simulink model "Cascata_piu_anelli"  (R2023b)
settings: Solver=VariableStepAuto  StartTime=0.0  StopTime=4  RelTol=1e-3
values from neighbouring files (symbols this model uses):
  den = [1 437.9395]    [controllore_piu_anelli.m]
  den_ext = [1 0]    [controllore_piu_anelli.m]
  Gdclose = Gdclose{1}    [controllore_piu_anelli.m]
  Gden = Gden{1}    [controllore_piu_anelli.m]
  Gnclose = Gnclose{1}    [controllore_piu_anelli.m]
  Gnum = Gnum{1}    [controllore_piu_anelli.m]
  num = [916.9165 8.0682e+04]    [controllore_piu_anelli.m]
  num_ext = [0.0081249 23.37*0.0081249]    [controllore_piu_anelli.m]
  ueq = 15/Rtot    [controllore_piu_anelli.m]
  x1_eq = 0.0044    [Controllo_un_anello_v2.m]    (also in Controllore_testato.m)
undefined symbols (not defined in the file or in its folder): ki, kp, Lc, Rtot
libraries: slpidlib x3
settings Model: Creator=lollo  LastModifiedBy=lollo

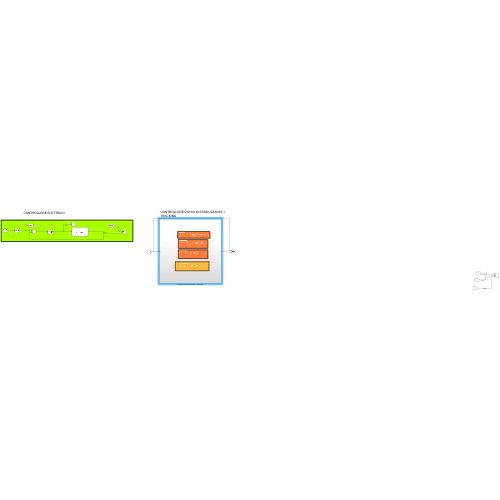
[thumbnail: Simulink's stored preview of the top-level diagram]
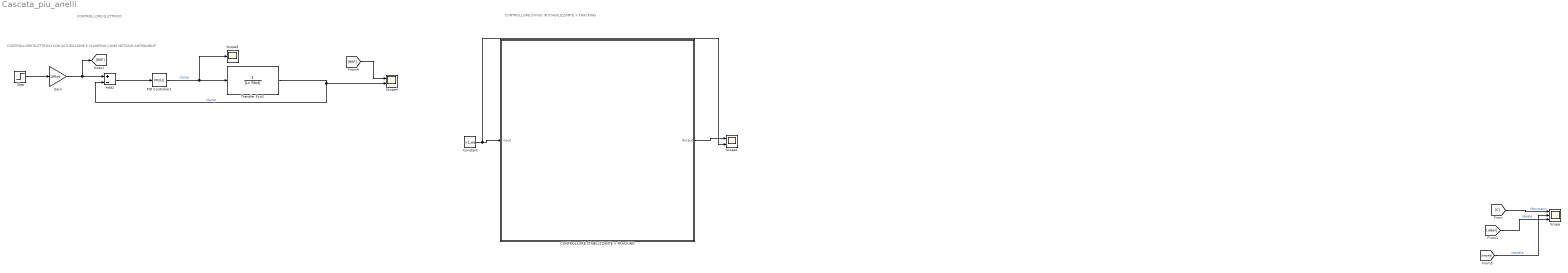
== system Cascata_piu_anelli ==
  note: CONTROLLORE ELETTRICO
  note: CONTROLLORE DIVISO IN STABILIZZANTE + TRACKING
  note: CONTROLLORE ELETTRICO CON SATURAZIONE E CLAMPING COME METODO ANTIWINDUP
  Add2 : Sum  Inputs=+-
  CONTROLLORE STABILIZZANTE + TRACKING : Subsystem
  Constant : Constant  Value=x1_eq
  Gain : Gain  Gain=1/Rtot
  PID Controller1 : slpidlib/PID Controller  Controller=PID  Form=Parallel  TimeDomain=Continuous-time  UseExternalTs=off  SampleTime=-1  IntegratorMethod=Forward Euler  FilterMethod=Forward Euler  ControllerParametersSource=internal  P=kp  I=ki  UseKiTs=off  D=0  N=100  UseFilter=on  TunerSelectOption=Transfer Function Based (PID Tuner App)  InitialConditionSource=internal  InitialConditionForIntegrator=0  InitialConditionForFilter=0  DifferentiatorICPrevScaledInput=0  ExternalReset=none  TrackingMode=off  Kt=1  LimitOutput=on  SatLimitsSource=internal  UpperSaturationLimit=23  LowerSaturationLimit=-23  LinearizeAsGain=on  AntiWindupMode=clamping  Kb=1  LimitIntegrator=off  UpperIntegratorSaturationLimit=inf  LowerIntegratorSaturationLimit=-inf  POutMin=[]  POutMax=[]  IOutMin=[]  IOutMax=[]  DOutMin=[]  DOutMax=[]  NOutMin=[]  NOutMax=[]  SumOutMin=[]  SumOutMax=[]  SaturationOutMin=[]  SaturationOutMax=[]  PParamMin=[]  PParamMax=[]  IParamMin=[]  IParamMax=[]  DParamMin=[]  DParamMax=[]  NParamMin=[]  NParamMax=[]  KbParamMin=[]  KbParamMax=[]  KtParamMin=[]  KtParamMax=[]  KbOutMin=[]  KbOutMax=[]  KtOutMin=[]  KtOutMax=[]  IntegratorOutMin=[]  IntegratorOutMax=[]  FilterOutMin=[]  FilterOutMax=[]  SumI1OutMin=[]  SumI1OutMax=[]  SumI2OutMin=[]  SumI2OutMax=[]  SumI3OutMin=[]  SumI3OutMax=[]  SumI4OutMin=[]  SumI4OutMax=[]  SumDOutMin=[]  SumDOutMax=[]  DifferentiatorOutMin=[]  DifferentiatorOutMax=[]  FilterDiffOutCoefMin=[]  FilterDiffOutCoefMax=[]  ReciprocalOutMin=[]  ReciprocalOutMax=[]  SumDenOutMin=[]  SumDenOutMax=[]  SumNumOutMin=[]  SumNumOutMax=[]  DivideOutMin=[]  DivideOutMax=[]  UdiffTsProdOutMin=[]  UdiffTsProdOutMax=[]  NTsProdOutMin=[]  NTsProdOutMax=[]  UintegralTsProdOutMin=[]  UintegralTsProdOutMax=[]  UngainTsProdOutMin=[]  UngainTsProdOutMax=[]  ClampingZeroOutDataTypeStr=Inherit: Inherit via back propagation  ClampingZeroOutMin=[]  ClampingZeroOutMax=[]  FilterDenConstantOutDataTypeStr=Inherit: Inherit via back propagation  FilterDenConstantOutMin=[]  FilterDenConstantOutMax=[]  PCopyOutDataTypeStr=Inherit: Inherit via back propagation  PCopyOutMin=[]  PCopyOutMax=[]  NCopyOutDataTypeStr=Inherit: Inherit via back propagation  NCopyOutMin=[]  NCopyOutMax=[]  IntegratorContinuousStateAttributes=''  IntegratorStateMustResolveToSignalObject=off  IntegratorRTWStateStorageClass=Auto  FilterContinuousStateAttributes=''  FilterStateMustResolveToSignalObject=off  FilterRTWStateStorageClass=Auto  ParallelPVariant=InternalParameters  IdealPVariant=Disabled  IVariant=InternalParameters  DVariant=InternalParameters  IntegratorVariant=Continuous  SatVariant=Enabled  AWVariant=ContClampingParallel  PCopyVariant=Disabled  TRVariant=Disabled  FdbkBlocksVariant=Forward  IdealPFdbkVariant=Disabled  SatFdbkVariant=Disabled  DerivativeFilterVariant=ContFilter  NVariant=InternalParameters  NCopyVariant=Disabled  FilterICVariant=InternalICsFilter  IntegratorICVariant=InternalICs  ExternalResetVariant=Disabled  TRSumVariant=Passthrough  SumFdbkVariant=Disabled  SumVariant=Sum_PID  TsampFilterVariant=InternalTs  TsampNgainVariant=Passthrough  TsampIntegralVariant=Disabled_SignalSpec  ExternalSaturationOutDataTypeStr=Inherit: Same as second input
  Scope : Scope  NumInputPorts=3
  Scope1 : Scope  NumInputPorts=2
  Scope4 : Scope  NumInputPorts=2
  Scope5 : Scope
  Step : Step  Time=0  After=10  SampleTime=0
  Transfer Fcn2 : TransferFcn  Denominator=[Lc Rtot]
  wires:
  Add2/1 -> PID Controller1/1
  PID Controller1/1 -> Scope5/1, Transfer Fcn2/1  "clamp"
  Transfer Fcn2/1 -> Scope4/2, Add2/2  "clamp"
  Step/1 -> Gain/1
  [REF] -> Scope4/1
  [C] -> Scope/1  "riferimenti"
  [ideal] -> Scope/3  "ideale"
  [cascata] -> Scope/2  "cascata"
  Gain/1 -> [REF], Add2/1
  Constant/1 -> Scope1/2, CONTROLLORE STABILIZZANTE + TRACKING/1(Input)
  CONTROLLORE STABILIZZANTE + TRACKING/1(Output) -> Scope1/1

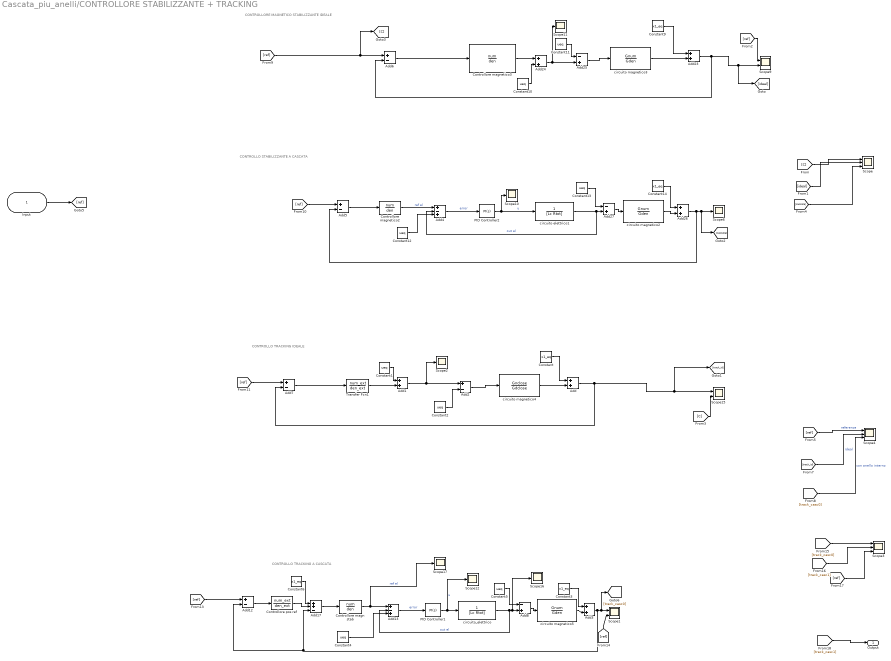
== system Cascata_piu_anelli/CONTROLLORE STABILIZZANTE + TRACKING ==
  note: CONTROLLO STABILIZZANTE A CASCATA
  note: CONTROLLORE MAGNETICO STABILIZZANTE IDEALE
  note: CONTROLLO TRACKING IDEALE
  note: CONTROLLO TRACKING A CASCATA
  Input : Inport
  Add{,1,3,23..24,26} (6 alike) : Sum
  Add{2,5..7,12} (5 alike) : Sum  Inputs=+-
  Add13 : Sum  Inputs=+-+
  Add17 : Sum  Inputs=++-
  Add25 : Sum  Inputs=-+
  Add27 : Sum  Inputs=-+
  Add4 : Sum  Inputs=+-+
  Add8 : Sum  Inputs=-+
  Constant{,3,6,9,14} (5 alike) : Constant  Value=x1_eq
  Constant{1..2,4..5,10..13} (8 alike) : Constant  Value=ueq
  Controllore magn stab : TransferFcn  Numerator=num  Denominator=den
  Controllore magnetico2 : TransferFcn  Numerator=num  Denominator=den
  Controllore magnetico3 : TransferFcn  Numerator=num  Denominator=den
  Controllore pos ref : TransferFcn  Numerator=num_ext  Denominator=den_ext
  PID Controller1 : slpidlib/PID Controller  Controller=PI  Form=Parallel  TimeDomain=Continuous-time  UseExternalTs=off  SampleTime=-1  IntegratorMethod=Forward Euler  FilterMethod=Forward Euler  ControllerParametersSource=internal  P=kp  I=ki  UseKiTs=off  D=0  N=100  UseFilter=on  TunerSelectOption=Transfer Function Based (PID Tuner App)  InitialConditionSource=internal  InitialConditionForIntegrator=0  InitialConditionForFilter=0  DifferentiatorICPrevScaledInput=0  ExternalReset=none  TrackingMode=off  Kt=1  LimitOutput=off  SatLimitsSource=internal  UpperSaturationLimit=23  LowerSaturationLimit=-23  LinearizeAsGain=on  AntiWindupMode=clamping  Kb=1  LimitIntegrator=off  UpperIntegratorSaturationLimit=inf  LowerIntegratorSaturationLimit=-inf  POutMin=[]  POutMax=[]  IOutMin=[]  IOutMax=[]  DOutMin=[]  DOutMax=[]  NOutMin=[]  NOutMax=[]  SumOutMin=[]  SumOutMax=[]  SaturationOutMin=[]  SaturationOutMax=[]  PParamMin=[]  PParamMax=[]  IParamMin=[]  IParamMax=[]  DParamMin=[]  DParamMax=[]  NParamMin=[]  NParamMax=[]  KbParamMin=[]  KbParamMax=[]  KtParamMin=[]  KtParamMax=[]  KbOutMin=[]  KbOutMax=[]  KtOutMin=[]  KtOutMax=[]  IntegratorOutMin=[]  IntegratorOutMax=[]  FilterOutMin=[]  FilterOutMax=[]  SumI1OutMin=[]  SumI1OutMax=[]  SumI2OutMin=[]  SumI2OutMax=[]  SumI3OutMin=[]  SumI3OutMax=[]  SumI4OutMin=[]  SumI4OutMax=[]  SumDOutMin=[]  SumDOutMax=[]  DifferentiatorOutMin=[]  DifferentiatorOutMax=[]  FilterDiffOutCoefMin=[]  FilterDiffOutCoefMax=[]  ReciprocalOutMin=[]  ReciprocalOutMax=[]  SumDenOutMin=[]  SumDenOutMax=[]  SumNumOutMin=[]  SumNumOutMax=[]  DivideOutMin=[]  DivideOutMax=[]  UdiffTsProdOutMin=[]  UdiffTsProdOutMax=[]  NTsProdOutMin=[]  NTsProdOutMax=[]  UintegralTsProdOutMin=[]  UintegralTsProdOutMax=[]  UngainTsProdOutMin=[]  UngainTsProdOutMax=[]  ClampingZeroOutDataTypeStr=Inherit: Inherit via back propagation  ClampingZeroOutMin=[]  ClampingZeroOutMax=[]  FilterDenConstantOutDataTypeStr=Inherit: Inherit via back propagation  FilterDenConstantOutMin=[]  FilterDenConstantOutMax=[]  PCopyOutDataTypeStr=Inherit: Inherit via back propagation  PCopyOutMin=[]  PCopyOutMax=[]  NCopyOutDataTypeStr=Inherit: Inherit via back propagation  NCopyOutMin=[]  NCopyOutMax=[]  IntegratorContinuousStateAttributes=''  IntegratorStateMustResolveToSignalObject=off  IntegratorRTWStateStorageClass=Auto  FilterContinuousStateAttributes=''  FilterStateMustResolveToSignalObject=off  FilterRTWStateStorageClass=Auto  ParallelPVariant=InternalParameters  IdealPVariant=Disabled  IVariant=InternalParameters  DVariant=Disabled  IntegratorVariant=Continuous  SatVariant=Disabled  AWVariant=Passthrough  PCopyVariant=Disabled  TRVariant=Disabled  FdbkBlocksVariant=Forward  IdealPFdbkVariant=Disabled  SatFdbkVariant=Disabled  DerivativeFilterVariant=Disabled  NVariant=Disabled  NCopyVariant=Disabled_SignalSpec  FilterICVariant=Disabled  IntegratorICVariant=InternalICs  ExternalResetVariant=Disabled  TRSumVariant=Passthrough  SumFdbkVariant=Disabled  SumVariant=Sum_PI  TsampFilterVariant=InternalTs  TsampNgainVariant=Passthrough  TsampIntegralVariant=Disabled_SignalSpec  ExternalSaturationOutDataTypeStr=Inherit: Same as second input
  PID Controller2 : slpidlib/PID Controller  Controller=PI  Form=Parallel  TimeDomain=Continuous-time  UseExternalTs=off  SampleTime=-1  IntegratorMethod=Forward Euler  FilterMethod=Forward Euler  ControllerParametersSource=internal  P=kp  I=ki  UseKiTs=off  D=0  N=100  UseFilter=on  TunerSelectOption=Transfer Function Based (PID Tuner App)  InitialConditionSource=internal  InitialConditionForIntegrator=0  InitialConditionForFilter=0  DifferentiatorICPrevScaledInput=0  ExternalReset=none  TrackingMode=off  Kt=1  LimitOutput=off  SatLimitsSource=internal  UpperSaturationLimit=23  LowerSaturationLimit=-23  LinearizeAsGain=on  AntiWindupMode=clamping  Kb=1  LimitIntegrator=off  UpperIntegratorSaturationLimit=inf  LowerIntegratorSaturationLimit=-inf  POutMin=[]  POutMax=[]  IOutMin=[]  IOutMax=[]  DOutMin=[]  DOutMax=[]  NOutMin=[]  NOutMax=[]  SumOutMin=[]  SumOutMax=[]  SaturationOutMin=[]  SaturationOutMax=[]  PParamMin=[]  PParamMax=[]  IParamMin=[]  IParamMax=[]  DParamMin=[]  DParamMax=[]  NParamMin=[]  NParamMax=[]  KbParamMin=[]  KbParamMax=[]  KtParamMin=[]  KtParamMax=[]  KbOutMin=[]  KbOutMax=[]  KtOutMin=[]  KtOutMax=[]  IntegratorOutMin=[]  IntegratorOutMax=[]  FilterOutMin=[]  FilterOutMax=[]  SumI1OutMin=[]  SumI1OutMax=[]  SumI2OutMin=[]  SumI2OutMax=[]  SumI3OutMin=[]  SumI3OutMax=[]  SumI4OutMin=[]  SumI4OutMax=[]  SumDOutMin=[]  SumDOutMax=[]  DifferentiatorOutMin=[]  DifferentiatorOutMax=[]  FilterDiffOutCoefMin=[]  FilterDiffOutCoefMax=[]  ReciprocalOutMin=[]  ReciprocalOutMax=[]  SumDenOutMin=[]  SumDenOutMax=[]  SumNumOutMin=[]  SumNumOutMax=[]  DivideOutMin=[]  DivideOutMax=[]  UdiffTsProdOutMin=[]  UdiffTsProdOutMax=[]  NTsProdOutMin=[]  NTsProdOutMax=[]  UintegralTsProdOutMin=[]  UintegralTsProdOutMax=[]  UngainTsProdOutMin=[]  UngainTsProdOutMax=[]  ClampingZeroOutDataTypeStr=Inherit: Inherit via back propagation  ClampingZeroOutMin=[]  ClampingZeroOutMax=[]  FilterDenConstantOutDataTypeStr=Inherit: Inherit via back propagation  FilterDenConstantOutMin=[]  FilterDenConstantOutMax=[]  PCopyOutDataTypeStr=Inherit: Inherit via back propagation  PCopyOutMin=[]  PCopyOutMax=[]  NCopyOutDataTypeStr=Inherit: Inherit via back propagation  NCopyOutMin=[]  NCopyOutMax=[]  IntegratorContinuousStateAttributes=''  IntegratorStateMustResolveToSignalObject=off  IntegratorRTWStateStorageClass=Auto  FilterContinuousStateAttributes=''  FilterStateMustResolveToSignalObject=off  FilterRTWStateStorageClass=Auto  ParallelPVariant=InternalParameters  IdealPVariant=Disabled  IVariant=InternalParameters  DVariant=Disabled  IntegratorVariant=Continuous  SatVariant=Disabled  AWVariant=Passthrough  PCopyVariant=Disabled  TRVariant=Disabled  FdbkBlocksVariant=Forward  IdealPFdbkVariant=Disabled  SatFdbkVariant=Disabled  DerivativeFilterVariant=Disabled  NVariant=Disabled  NCopyVariant=Disabled_SignalSpec  FilterICVariant=Disabled  IntegratorICVariant=InternalICs  ExternalResetVariant=Disabled  TRSumVariant=Passthrough  SumFdbkVariant=Disabled  SumVariant=Sum_PI  TsampFilterVariant=InternalTs  TsampNgainVariant=Passthrough  TsampIntegralVariant=Disabled_SignalSpec  ExternalSaturationOutDataTypeStr=Inherit: Same as second input
  Scope : Scope  NumInputPorts=3
  Scope1 : Scope  NumInputPorts=2
  Scope{2,6,10..12,16..17} (7 alike) : Scope
  Scope15 : Scope  NumInputPorts=2
  Scope3 : Scope  NumInputPorts=3
  Scope4 : Scope  NumInputPorts=3
  Scope9 : Scope  NumInputPorts=2
  Transfer Fcn1 : TransferFcn  Numerator=num_ext  Denominator=den_ext
  circuito elettrico1 : TransferFcn  Denominator=[Lc Rtot]
  circuito magnetico2 : TransferFcn  Numerator=Gnum  Denominator=Gden
  circuito magnetico3 : TransferFcn  Numerator=Gnum  Denominator=Gden
  circuito magnetico4 : TransferFcn  Numerator=Gnclose  Denominator=Gdclose
  circuito magnetico5 : TransferFcn  Numerator=Gnum  Denominator=Gden
  circuito_elettrico : TransferFcn  Denominator=[Lc Rtot]
  Output : Outport
  wires:
  circuito elettrico1/1 -> Add27/2, Add4/2  "out el"
  Add4/1 -> PID Controller2/1  "error"
  Controllore magnetico2/1 -> Add4/1  "ref el"
  Add5/1 -> Controllore magnetico2/1
  [ref] -> Add5/1
  PID Controller2/1 -> Scope10/1, circuito elettrico1/1  "u"
  Add6/1 -> Controllore magnetico3/1
  [ref] -> [C], Add6/1
  [ref] -> Scope9/1
  [ref] -> Add7/1
  [C] -> Scope15/2
  Add7/1 -> Transfer Fcn1/1
  [C] -> Scope/1
  [ideal] -> Scope/2
  [cascata] -> Scope/3
  [ref] -> Scope4/1  "reference"
  [track_id] -> Scope4/2  "ideal"
  [track_casc0] -> Scope4/3  "con anello interno"
  Input/1 -> [ref]
  [ref] -> Add12/1
  Controllore magn stab/1 -> Scope17/1, Add13/1  "ref el"
  circuito_elettrico/1 -> Add8/2, Scope16/1, Add13/2  "out el"
  Controllore pos ref/1 -> Add17/2
  Add12/1 -> Controllore pos ref/1
  [ref] -> Scope1/2
  Add17/1 -> Controllore magn stab/1
  PID Controller1/1 -> Scope12/1, circuito_elettrico/1  "u"
  Add13/1 -> PID Controller1/1  "error"
  [track_casc0] -> Scope3/1
  [track_casc1] -> Scope3/2
  [ref] -> Scope3/3
  [track_casc1] -> Output/1
  circuito magnetico3/1 -> Add23/2
  Add23/1 -> Add6/2, [ideal], Scope9/2
  Constant9/1 -> Add23/1
  Constant10/1 -> Add24/2
  Controllore magnetico3/1 -> Add24/1
  Add24/1 -> Scope11/1, Add25/2
  Constant11/1 -> Add25/1
  Add25/1 -> circuito magnetico3/1
  Constant12/1 -> Add4/3
  Add27/1 -> circuito magnetico2/1
  Constant13/1 -> Add27/1
  circuito magnetico2/1 -> Add26/2
  Constant14/1 -> Add26/1
  Add26/1 -> Add5/2, [cascata], Scope6/1
  circuito magnetico4/1 -> Add/2
  Constant/1 -> Add/1
  Add/1 -> Add7/2, [track_id], Scope15/1
  Transfer Fcn1/1 -> Add1/2
  Add2/1 -> circuito magnetico4/1
  Constant1/1 -> Add1/1
  Constant2/1 -> Add2/2
  Add1/1 -> Scope2/1, Add2/1
  Add3/1 -> Add17/3, Add12/2, [track_casc0], Scope1/1
  circuito magnetico5/1 -> Add3/2
  Constant3/1 -> Add3/1
  Constant4/1 -> Add13/3
  Add8/1 -> circuito magnetico5/1
  Constant5/1 -> Add8/1
  Constant6/1 -> Add17/1
